simulink model "H250Model2019b"  (R2019b)
settings: Solver=ode4  StartTime=0.0  StopTime=inf  FixedStep=Ts  RelTol=1e-3
values from neighbouring files (symbols this model uses):
  ModelFail_env_P_wind = [0 0 0]    [F450DegradedParamInit.m]    (also in H250DegradedParamInit.m; H250ModelParam4S.m; H333DegradedParamInit4S.m)
  ModelFail_motor_isEnable = 0    [F450DegradedParamInit.m]    (also in H250DegradedParamInit.m; H250ModelParam4S.m; H333DegradedParamInit4S.m)
  ModelFail_motor_kCt = [1 1 1 1 1 1 1 1]    [F450DegradedParamInit.m]    (also in H250DegradedParamInit.m; H250ModelParam4S.m; H333DegradedParamInit4S.m)
  ModelFail_motor_kTc = [1 1 1 1 1 1 1 1]    [F450DegradedParamInit.m]    (also in H250DegradedParamInit.m; H250ModelParam4S.m; H333DegradedParamInit4S.m)
  ModelFail_motor_kw = [1 1 1 1 1 1 1 1]    [F450DegradedParamInit.m]    (also in H250DegradedParamInit.m; H250ModelParam4S.m; H333DegradedParamInit4S.m)
  ModelInit_motorInitRate = 0    [F450DegradedParamInit.m]    (also in H250DegradedParamInit.m; H250ModelParam4S.m; H333DegradedParamInit4S.m)
  ModelParam_Airframe_CMP = [0 0 0]    [F450DegradedParamInit.m]    (also in H250DegradedParamInit.m; H250ModelParam4S.m; H333DegradedParamInit4S.m)
  ModelParam_Airframe_J = [0.0194 0 0;0 0.0194 0;0 0 0.0291]    [F450DegradedParamInit.m]    (also in H250DegradedParamInit.m = [0.0056 0 0;0 0.0056 0;0 0 0.0104]; H250ModelParam4S.m = [0.0056 0 0;0 0.0056 0;0 0 0.0104]; H333DegradedParamInit4S.m = [0.012 0 0;0 0.012 0;0 0 0.02])
  ModelParam_Airframe_m = 1.31    [F450DegradedParamInit.m]    (also in H250DegradedParamInit.m = 0.752; H250ModelParam4S.m = 0.752; H333DegradedParamInit4S.m = 1.13)
  ModelParam_envAltitude = 0    [F450DegradedParamInit.m]    (also in H250DegradedParamInit.m; H250ModelParam4S.m; H333DegradedParamInit4S.m)
  ModelParam_envC_d = 0.055    [F450DegradedParamInit.m]    (also in H250DegradedParamInit.m; H250ModelParam4S.m; H333DegradedParamInit4S.m)
  ModelParam_envC_md = [0.001 0.001 0.00058]    [F450DegradedParamInit.m]    (also in H250DegradedParamInit.m = [0.001 0.001 0.00040]; H250ModelParam4S.m = [0.001 0.001 0.00040]; H333DegradedParamInit4S.m = [0.001 0.001 0.0002])
  ModelParam_GPSEphFinal = 0.3    [F450DegradedParamInit.m]    (also in H250DegradedParamInit.m; H250ModelParam4S.m; H333DegradedParamInit4S.m)
  ModelParam_GPSEpvFinal = 0.4    [F450DegradedParamInit.m]    (also in H250DegradedParamInit.m; H250ModelParam4S.m; H333DegradedParamInit4S.m)
  ModelParam_GPSFix3DFix = 3    [F450DegradedParamInit.m]    (also in H250DegradedParamInit.m; H250ModelParam4S.m; H333DegradedParamInit4S.m)
  ModelParam_GPSSatsVisible = 10    [F450DegradedParamInit.m]    (also in H250DegradedParamInit.m; H250ModelParam4S.m; H333DegradedParamInit4S.m)
  ModelParam_motorCr = 842.1    [F450DegradedParamInit.m]    (also in H250DegradedParamInit.m = 0; H250ModelParam4S.m = 0; H333DegradedParamInit4S.m = 0)
  ModelParam_motorFitType = 1    [F450DegradedParamInit.m]    (also in H250DegradedParamInit.m = 2; H250ModelParam4S.m = 2; H333DegradedParamInit4S.m = 2)
  ModelParam_motorJm = 0.0000687    (= 6.87e-05)    [F450DegradedParamInit.m]    (also in H250DegradedParamInit.m = 8.8493e-06; H250ModelParam4S.m = 8.8493e-06; H333DegradedParamInit4S.m = 8.8493e-06)
  ModelParam_motorMinThr = 0.05    [F450DegradedParamInit.m]    (also in H250DegradedParamInit.m = 0.148; H250ModelParam4S.m = 0.148; H333DegradedParamInit4S.m = 0.11)
  ModelParam_motorRateCurveCoeffi = [0 0 0]    [F450DegradedParamInit.m]    (also in H250DegradedParamInit.m = [-1364 3870 -372.4]; H250ModelParam4S.m = [-2143 5113 -458.4]; H333DegradedParamInit4S.m = [-1057 2662 -94.98])
  ModelParam_motorTc = 0.0214    [F450DegradedParamInit.m]    (also in H250DegradedParamInit.m = 0.035; H250ModelParam4S.m = 0.032; H333DegradedParamInit4S.m = 0.035)
  ModelParam_motorWb = 0    [F450DegradedParamInit.m]    (also in H250DegradedParamInit.m; H250ModelParam4S.m; H333DegradedParamInit4S.m)
  ModelParam_NoiseVarAcc0 = [0.1 0.1 0.1]    [F450DegradedParamInit.m]    (also in H250DegradedParamInit.m; H250ModelParam4S.m = [0.01 0.01 0.01]; H333DegradedParamInit4S.m)
  ModelParam_NoiseVarAcc1 = [0.1 0.1 0.1]    [F450DegradedParamInit.m]    (also in H250DegradedParamInit.m; H250ModelParam4S.m = [0.01 0.01 0.01]; H333DegradedParamInit4S.m)
  ModelParam_NoiseVarGPS_P0 = [1e-5 1e-5 1e-5]    [F450DegradedParamInit.m]    (also in H250DegradedParamInit.m; H250ModelParam4S.m; H333DegradedParamInit4S.m)
  ModelParam_NoiseVarGPS_V0 = [1e-5 1e-5 1e-5]    [F450DegradedParamInit.m]    (also in H250DegradedParamInit.m; H250ModelParam4S.m; H333DegradedParamInit4S.m)
  ModelParam_NoiseVarGyro0 = [0.0005 0.0005 0.0005]    [F450DegradedParamInit.m]    (also in H250DegradedParamInit.m; H250ModelParam4S.m; H333DegradedParamInit4S.m)
  ModelParam_NoiseVarGyro1 = [0.004 0.004 0.004]    [F450DegradedParamInit.m]    (also in H250DegradedParamInit.m; H250ModelParam4S.m; H333DegradedParamInit4S.m)
  ModelParam_NoiseVarMag0 = [0.000002 0.000002 0.000002]    [F450DegradedParamInit.m]    (also in H250DegradedParamInit.m; H250ModelParam4S.m; H333DegradedParamInit4S.m)
  ModelParam_NoiseVarMag1 = [0.0001 0.0001 0.0001]    [F450DegradedParamInit.m]    (also in H250DegradedParamInit.m; H250ModelParam4S.m; H333DegradedParamInit4S.m)
  ModelParam_PositionAcc0 = [0.071  0  -0.1365]    [F450DegradedParamInit.m]    (also in H250DegradedParamInit.m; H250ModelParam4S.m; H333DegradedParamInit4S.m)
  ModelParam_PositionAcc1 = [0.071  0  -0.1365]    [F450DegradedParamInit.m]    (also in H250DegradedParamInit.m; H250ModelParam4S.m; H333DegradedParamInit4S.m)
  ModelParam_rotorCt = 1.681e-05    [F450DegradedParamInit.m]    (also in H250DegradedParamInit.m = 1.448e-06; H250ModelParam4S.m = 1.345e-06; H333DegradedParamInit4S.m = 7.586e-06)
  ModelParam_WalkNoiseVarAcc0 = [0.001 0.001 0.001]    [F450DegradedParamInit.m]    (also in H250DegradedParamInit.m; H250ModelParam4S.m; H333DegradedParamInit4S.m)
  ModelParam_WalkNoiseVarAcc1 = [0.001 0.001 0.001]    [F450DegradedParamInit.m]    (also in H250DegradedParamInit.m; H250ModelParam4S.m; H333DegradedParamInit4S.m)
  ModelParam_WalkNoiseVarGPS_P0 = [0.01 0.01 0.01]    [F450DegradedParamInit.m]    (also in H250DegradedParamInit.m; H250ModelParam4S.m = [0 0 0]; H333DegradedParamInit4S.m)
  ModelParam_WalkNoiseVarGPS_V0 = [0.01 0.01 0.01]    [F450DegradedParamInit.m]    (also in H250DegradedParamInit.m; H250ModelParam4S.m = [0 0 0]; H333DegradedParamInit4S.m)
  ModelParam_WalkNoiseVarGyro0 = [0.00004 0.00004 0.00004]    [F450DegradedParamInit.m]    (also in H250DegradedParamInit.m; H250ModelParam4S.m; H333DegradedParamInit4S.m)
  ModelParam_WalkNoiseVarGyro1 = [0.00004 0.00004 0.00004]    [F450DegradedParamInit.m]    (also in H250DegradedParamInit.m; H250ModelParam4S.m; H333DegradedParamInit4S.m)
  ModelParam_WalkNoiseVarMag0 = [0.000001 0.000001 0.000001]    [F450DegradedParamInit.m]    (also in H250DegradedParamInit.m; H250ModelParam4S.m; H333DegradedParamInit4S.m)
  ModelParam_WalkNoiseVarMag1 = [0.000001 0.000001 0.000001]    [F450DegradedParamInit.m]    (also in H250DegradedParamInit.m; H250ModelParam4S.m; H333DegradedParamInit4S.m)
  MulticopterLayoutConfig = 1    [F450DegradedParamInit.m]    (also in H250DegradedParamInit.m = 6; H250ModelParam4S.m = 7; H333DegradedParamInit4S.m = 8)
  RflySimDisplayUAVType = 3    [F450DegradedParamInit.m]    (also in H250DegradedParamInit.m; H250ModelParam4S.m; H333DegradedParamInit4S.m)
  Ts = 1/1000    (= 0.001)    [F450DegradedParamInit.m]    (also in H250DegradedParamInit.m; H250ModelParam4S.m; H333DegradedParamInit4S.m)
undefined symbols (not defined in the file or in its folder): Earth, WGS84
libraries: aerolibnav x5, aerolibtransform2 x3, sharedtransform x3, aerolibutil x2, sharedutil x1, shared6dof x1, aerolibasang x1, aerolibatmos2 x1, aerolibconvert2 x1
(part 2 of 3)

== system H250Model2019b/ESC&Motor Model/MotorNonlinearDynamic4 ==
  Throttle : Inport
  BatteryEfficiency : Inport  Port=2  Unit=V
  k_omage : Inport  Port=3
  k_Tc : Inport  Port=4
  k_ct : Inport  Port=5
  ESC_MotorSteadyState : MATLAB Function  TreatAsAtomicUnit=on  mask{MotorMinThr=MotorMinThr}
      mask prompts: MotorMinThr "Minimum Throttle"
  ModelInit_motorInitRate : Constant  Value=motorInitRate
  ModelParam_motorCr : Constant  Value=motorCr
  ModelParam_motorFitType : Constant  Value=motorFitType
  ModelParam_motorRateCurveCoeffi : Constant  Value=motorRateCurveCoeffi
  ModelParam_motorTc : Constant  Value=motorTc
  ModelParam_motorWb : Constant  Value=motorWb
  ModelParam_rotorCt : Constant  Value=rotorCt
  MotorDynamic : Subsystem
      mask Display:
      | port_label('input', 1, '\varpi_{ss}(rad/s)', 'texmode', 'on');
      | port_label('input', 2, '\varpi_{0}(rad/s)', 'texmode', 'on');
      | port_label('input', 3, 'T_{c}(s)', 'texmode', 'on');
      | port_label('output', 1, '\varpi(rad/s)', 'texmode', 'on');
  Product{,1..3} (4 alike) : Product
  Square : Math  Operator=square  SaturateOnIntegerOverflow=on
  T : Outport  Unit=N
  MotorRate : Outport  Port=2  Unit=rad/s
  wires:
  ModelParam_motorFitType/1 -> ESC_MotorSteadyState/6(MotorFitType)
  ModelParam_motorRateCurveCoeffi/1 -> ESC_MotorSteadyState/5(MotorRateCurveCoeffi)
  k_ct/1 -> Product1/2
  k_Tc/1 -> Product2/2
  k_omage/1 -> Product3/1
  Product3/1 -> MotorDynamic/1(ReferenceRate)
  Product2/1 -> MotorDynamic/3(MotorTimeConstant)
  Product1/1 -> Product/2
  BatteryEfficiency/1 -> ESC_MotorSteadyState/2(BatteryEfficiency)
  MotorDynamic/1(MotorRate) -> Square/1, MotorRate/1
  ModelParam_motorTc/1 -> Product2/1
  Square/1 -> Product/1
  ESC_MotorSteadyState/1(SteadyStateRate) -> Product3/2
  Product/1 -> T/1
  ModelParam_rotorCt/1 -> Product1/1
  ModelInit_motorInitRate/1 -> MotorDynamic/2(MotorInitRate)
  ModelParam_motorCr/1 -> ESC_MotorSteadyState/3(Cr)
  Throttle/1 -> ESC_MotorSteadyState/1(Throttle)
  ModelParam_motorWb/1 -> ESC_MotorSteadyState/4(Ratebias)

== system H250Model2019b/ESC&Motor Model/MotorNonlinearDynamic5 ==
  Throttle : Inport
  BatteryEfficiency : Inport  Port=2  Unit=V
  k_omage : Inport  Port=3
  k_Tc : Inport  Port=4
  k_ct : Inport  Port=5
  ESC_MotorSteadyState : MATLAB Function  TreatAsAtomicUnit=on  mask{MotorMinThr=MotorMinThr}
      mask prompts: MotorMinThr "Minimum Throttle"
  ModelInit_motorInitRate : Constant  Value=motorInitRate
  ModelParam_motorCr : Constant  Value=motorCr
  ModelParam_motorFitType : Constant  Value=motorFitType
  ModelParam_motorRateCurveCoeffi : Constant  Value=motorRateCurveCoeffi
  ModelParam_motorTc : Constant  Value=motorTc
  ModelParam_motorWb : Constant  Value=motorWb
  ModelParam_rotorCt : Constant  Value=rotorCt
  MotorDynamic : Subsystem
      mask Display:
      | port_label('input', 1, '\varpi_{ss}(rad/s)', 'texmode', 'on');
      | port_label('input', 2, '\varpi_{0}(rad/s)', 'texmode', 'on');
      | port_label('input', 3, 'T_{c}(s)', 'texmode', 'on');
      | port_label('output', 1, '\varpi(rad/s)', 'texmode', 'on');
  Product{,1..3} (4 alike) : Product
  Square : Math  Operator=square  SaturateOnIntegerOverflow=on
  T : Outport  Unit=N
  MotorRate : Outport  Port=2  Unit=rad/s
  wires:
  ModelParam_motorWb/1 -> ESC_MotorSteadyState/4(Ratebias)
  Throttle/1 -> ESC_MotorSteadyState/1(Throttle)
  ModelParam_motorCr/1 -> ESC_MotorSteadyState/3(Cr)
  ModelInit_motorInitRate/1 -> MotorDynamic/2(MotorInitRate)
  ModelParam_rotorCt/1 -> Product1/1
  Product/1 -> T/1
  ESC_MotorSteadyState/1(SteadyStateRate) -> Product3/2
  Square/1 -> Product/1
  ModelParam_motorTc/1 -> Product2/1
  MotorDynamic/1(MotorRate) -> MotorRate/1, Square/1
  BatteryEfficiency/1 -> ESC_MotorSteadyState/2(BatteryEfficiency)
  Product1/1 -> Product/2
  Product2/1 -> MotorDynamic/3(MotorTimeConstant)
  Product3/1 -> MotorDynamic/1(ReferenceRate)
  k_omage/1 -> Product3/1
  k_Tc/1 -> Product2/2
  k_ct/1 -> Product1/2
  ModelParam_motorRateCurveCoeffi/1 -> ESC_MotorSteadyState/5(MotorRateCurveCoeffi)
  ModelParam_motorFitType/1 -> ESC_MotorSteadyState/6(MotorFitType)

== system H250Model2019b/ESC&Motor Model/MotorNonlinearDynamic6 ==
  Throttle : Inport
  BatteryEfficiency : Inport  Port=2  Unit=V
  k_omage : Inport  Port=3
  k_Tc : Inport  Port=4
  k_ct : Inport  Port=5
  ESC_MotorSteadyState : MATLAB Function  TreatAsAtomicUnit=on  mask{MotorMinThr=MotorMinThr}
      mask prompts: MotorMinThr "Minimum Throttle"
  ModelInit_motorInitRate : Constant  Value=motorInitRate
  ModelParam_motorCr : Constant  Value=motorCr
  ModelParam_motorFitType : Constant  Value=motorFitType
  ModelParam_motorRateCurveCoeffi : Constant  Value=motorRateCurveCoeffi
  ModelParam_motorTc : Constant  Value=motorTc
  ModelParam_motorWb : Constant  Value=motorWb
  ModelParam_rotorCt : Constant  Value=rotorCt
  MotorDynamic : Subsystem
      mask Display:
      | port_label('input', 1, '\varpi_{ss}(rad/s)', 'texmode', 'on');
      | port_label('input', 2, '\varpi_{0}(rad/s)', 'texmode', 'on');
      | port_label('input', 3, 'T_{c}(s)', 'texmode', 'on');
      | port_label('output', 1, '\varpi(rad/s)', 'texmode', 'on');
  Product{,1..3} (4 alike) : Product
  Square : Math  Operator=square  SaturateOnIntegerOverflow=on
  T : Outport  Unit=N
  MotorRate : Outport  Port=2  Unit=rad/s
  wires:
  ModelParam_motorFitType/1 -> ESC_MotorSteadyState/6(MotorFitType)
  ModelParam_motorRateCurveCoeffi/1 -> ESC_MotorSteadyState/5(MotorRateCurveCoeffi)
  k_ct/1 -> Product1/2
  k_Tc/1 -> Product2/2
  k_omage/1 -> Product3/1
  Product3/1 -> MotorDynamic/1(ReferenceRate)
  Product2/1 -> MotorDynamic/3(MotorTimeConstant)
  Product1/1 -> Product/2
  BatteryEfficiency/1 -> ESC_MotorSteadyState/2(BatteryEfficiency)
  MotorDynamic/1(MotorRate) -> Square/1, MotorRate/1
  ModelParam_motorTc/1 -> Product2/1
  Square/1 -> Product/1
  ESC_MotorSteadyState/1(SteadyStateRate) -> Product3/2
  Product/1 -> T/1
  ModelParam_rotorCt/1 -> Product1/1
  ModelInit_motorInitRate/1 -> MotorDynamic/2(MotorInitRate)
  ModelParam_motorCr/1 -> ESC_MotorSteadyState/3(Cr)
  Throttle/1 -> ESC_MotorSteadyState/1(Throttle)
  ModelParam_motorWb/1 -> ESC_MotorSteadyState/4(Ratebias)

== system H250Model2019b/ESC&Motor Model/MotorNonlinearDynamic7 ==
  Throttle : Inport
  BatteryEfficiency : Inport  Port=2  Unit=V
  k_omage : Inport  Port=3
  k_Tc : Inport  Port=4
  k_ct : Inport  Port=5
  ESC_MotorSteadyState : MATLAB Function  TreatAsAtomicUnit=on  mask{MotorMinThr=MotorMinThr}
      mask prompts: MotorMinThr "Minimum Throttle"
  ModelInit_motorInitRate : Constant  Value=motorInitRate
  ModelParam_motorCr : Constant  Value=motorCr
  ModelParam_motorFitType : Constant  Value=motorFitType
  ModelParam_motorRateCurveCoeffi : Constant  Value=motorRateCurveCoeffi
  ModelParam_motorTc : Constant  Value=motorTc
  ModelParam_motorWb : Constant  Value=motorWb
  ModelParam_rotorCt : Constant  Value=rotorCt
  MotorDynamic : Subsystem
      mask Display:
      | port_label('input', 1, '\varpi_{ss}(rad/s)', 'texmode', 'on');
      | port_label('input', 2, '\varpi_{0}(rad/s)', 'texmode', 'on');
      | port_label('input', 3, 'T_{c}(s)', 'texmode', 'on');
      | port_label('output', 1, '\varpi(rad/s)', 'texmode', 'on');
  Product{,1..3} (4 alike) : Product
  Square : Math  Operator=square  SaturateOnIntegerOverflow=on
  T : Outport  Unit=N
  MotorRate : Outport  Port=2  Unit=rad/s
  wires:
  ModelParam_motorWb/1 -> ESC_MotorSteadyState/4(Ratebias)
  Throttle/1 -> ESC_MotorSteadyState/1(Throttle)
  ModelParam_motorCr/1 -> ESC_MotorSteadyState/3(Cr)
  ModelInit_motorInitRate/1 -> MotorDynamic/2(MotorInitRate)
  ModelParam_rotorCt/1 -> Product1/1
  Product/1 -> T/1
  ESC_MotorSteadyState/1(SteadyStateRate) -> Product3/2
  Square/1 -> Product/1
  ModelParam_motorTc/1 -> Product2/1
  MotorDynamic/1(MotorRate) -> MotorRate/1, Square/1
  BatteryEfficiency/1 -> ESC_MotorSteadyState/2(BatteryEfficiency)
  Product1/1 -> Product/2
  Product2/1 -> MotorDynamic/3(MotorTimeConstant)
  Product3/1 -> MotorDynamic/1(ReferenceRate)
  k_omage/1 -> Product3/1
  k_Tc/1 -> Product2/2
  k_ct/1 -> Product1/2
  ModelParam_motorRateCurveCoeffi/1 -> ESC_MotorSteadyState/5(MotorRateCurveCoeffi)
  ModelParam_motorFitType/1 -> ESC_MotorSteadyState/6(MotorFitType)

== system H250Model2019b/ESC&Motor Model/MotorNonlinearDynamic8 ==
  Throttle : Inport
  BatteryEfficiency : Inport  Port=2  Unit=V
  k_omage : Inport  Port=3
  k_Tc : Inport  Port=4
  k_ct : Inport  Port=5
  ESC_MotorSteadyState : MATLAB Function  TreatAsAtomicUnit=on  mask{MotorMinThr=MotorMinThr}
      mask prompts: MotorMinThr "Minimum Throttle"
  ModelInit_motorInitRate : Constant  Value=motorInitRate
  ModelParam_motorCr : Constant  Value=motorCr
  ModelParam_motorFitType : Constant  Value=motorFitType
  ModelParam_motorRateCurveCoeffi : Constant  Value=motorRateCurveCoeffi
  ModelParam_motorTc : Constant  Value=motorTc
  ModelParam_motorWb : Constant  Value=motorWb
  ModelParam_rotorCt : Constant  Value=rotorCt
  MotorDynamic : Subsystem
      mask Display:
      | port_label('input', 1, '\varpi_{ss}(rad/s)', 'texmode', 'on');
      | port_label('input', 2, '\varpi_{0}(rad/s)', 'texmode', 'on');
      | port_label('input', 3, 'T_{c}(s)', 'texmode', 'on');
      | port_label('output', 1, '\varpi(rad/s)', 'texmode', 'on');
  Product{,1..3} (4 alike) : Product
  Square : Math  Operator=square  SaturateOnIntegerOverflow=on
  T : Outport  Unit=N
  MotorRate : Outport  Port=2  Unit=rad/s
  wires:
  ModelParam_motorFitType/1 -> ESC_MotorSteadyState/6(MotorFitType)
  ModelParam_motorRateCurveCoeffi/1 -> ESC_MotorSteadyState/5(MotorRateCurveCoeffi)
  k_ct/1 -> Product1/2
  k_Tc/1 -> Product2/2
  k_omage/1 -> Product3/1
  Product3/1 -> MotorDynamic/1(ReferenceRate)
  Product2/1 -> MotorDynamic/3(MotorTimeConstant)
  Product1/1 -> Product/2
  BatteryEfficiency/1 -> ESC_MotorSteadyState/2(BatteryEfficiency)
  MotorDynamic/1(MotorRate) -> Square/1, MotorRate/1
  ModelParam_motorTc/1 -> Product2/1
  Square/1 -> Product/1
  ESC_MotorSteadyState/1(SteadyStateRate) -> Product3/2
  Product/1 -> T/1
  ModelParam_rotorCt/1 -> Product1/1
  ModelInit_motorInitRate/1 -> MotorDynamic/2(MotorInitRate)
  ModelParam_motorCr/1 -> ESC_MotorSteadyState/3(Cr)
  Throttle/1 -> ESC_MotorSteadyState/1(Throttle)
  ModelParam_motorWb/1 -> ESC_MotorSteadyState/4(Ratebias)

== system H250Model2019b/Environment Model/Ground Model ==
  m : Inport
  g : Inport  Port=2
  wb : Inport  Port=3
  Xe : Inport  Port=4
  Ve : Inport  Port=5
  EulerAng : Inport  Port=6
  DCM : Inport  Port=7
  TerrainZ : Inport  Port=8
  Direction Cosine Matrix to Quaternions : sharedtransform/Direction Cosine Matrix  to Quaternions  aMode=0  action=None  tolerance=eps(2)
      settings: SourceProductBaseCode=AE,PW,MT,UV,VE,VP
  Direction Cosine Matrix to Quaternions1 : sharedtransform/Direction Cosine Matrix  to Quaternions  aMode=aMode  action=None  tolerance=eps(2)
      settings: SourceProductBaseCode=AE,PW,MT,UV,VE,VP
  Euler to DCM : aerolibtransform2/Wind Angles to  Direction Cosine Matrix
      settings: SourceProductBaseCode=AE
  Ground Model : MATLAB Function  TreatAsAtomicUnit=on
  OnGroundFaceup : MATLAB Function  TreatAsAtomicUnit=on
  Product : Product  Multiplication=Matrix(*)
  Product1 : Product
  Quaternion Inverse : aerolibutil/Quaternion Inverse
  Quaternion Multiplication : aerolibutil/Quaternion Multiplication
  Terminator1 : Terminator
  F_Ground : Outport
  M_Ground : Outport  Port=2
  landed : Outport  Port=3
  wires:
  Xe/1 -> Ground Model/3(Xe)
  TerrainZ/1 -> Ground Model/6(terrainZ)
  OnGroundFaceup/1(y) -> Euler to DCM/1
  Ground Model/4(takeoff) -> Terminator1/1
  Direction Cosine Matrix to Quaternions1/1 -> Quaternion Inverse/1
  Quaternion Inverse/1 -> Quaternion Multiplication/1
  Direction Cosine Matrix to Quaternions/1 -> Quaternion Multiplication/2
  Ground Model/3(landed) -> landed/1
  Quaternion Multiplication/1 -> Ground Model/5(Quet)
  Ground Model/1(F1) -> Product/2
  Euler to DCM/1 -> Direction Cosine Matrix to Quaternions1/1
  Product1/1 -> Ground Model/1(mg)
  m/1 -> Product1/1
  Ground Model/2(M1) -> M_Ground/1
  wb/1 -> Ground Model/2(wb)
  Ve/1 -> Ground Model/4(Ve)
  g/1 -> Product1/2
  EulerAng/1 -> OnGroundFaceup/1(EulerAng)
  Product/1 -> F_Ground/1
  DCM/1 -> Direction Cosine Matrix to Quaternions/1, Product/1

== system H250Model2019b/Force and Moment Model/Allocation Model ==
  index : Inport
  MotorForces : Inport  Port=2
  Wb : Inport  Port=3
  o_m : Inport  Port=4
  MotorRate : Inport  Port=5
  3x3 Cross Product : sharedutil/3x3 Cross Product  aMode=aMode
      settings: SourceProductBaseCode=AE,PW,MT,UV,VE,VP
  Assignment : Assignment  IndexMode=Zero-based  DiagnosticForDimensions=Warning  IndexOptions=Index vector (dialog)  Indices=2  OutputSizes=1
  Constant : Constant  Value=[0;0;0]
  Demux : Demux  Outputs=[3 3]
  Efficiency Function : MATLAB Function  TreatAsAtomicUnit=on
  Gain : Gain  Gain=ModelParam_motorJm
  MatrixMultiply : Product  Multiplication=Matrix(*)
  MatrixMultiply1 : Product  Multiplication=Matrix(*)
  Reshape : Reshape  OutputDimensionality=Column vector (2-D)
  F : Outport
  M : Outport  Port=2
  M_G : Outport  Port=3
  wires:
  Demux/2 -> M/1
  MatrixMultiply/1 -> Demux/1
  MotorForces/1 -> MatrixMultiply/2
  Efficiency Function/1(EfficiencyMatrix) -> MatrixMultiply/1
  Demux/1 -> F/1
  o_m/1 -> Efficiency Function/2(o_m)
  index/1 -> Efficiency Function/1(index)
  Efficiency Function/2(RotorDirectionVector) -> MatrixMultiply1/1
  MotorRate/1 -> Reshape/1
  Constant/1 -> Assignment/1
  MatrixMultiply1/1 -> Gain/1
  Reshape/1 -> MatrixMultiply1/2
  Gain/1 -> Assignment/2
  Assignment/1 -> 3x3 Cross Product/2
  Wb/1 -> 3x3 Cross Product/1
  3x3 Cross Product/1 -> M_G/1

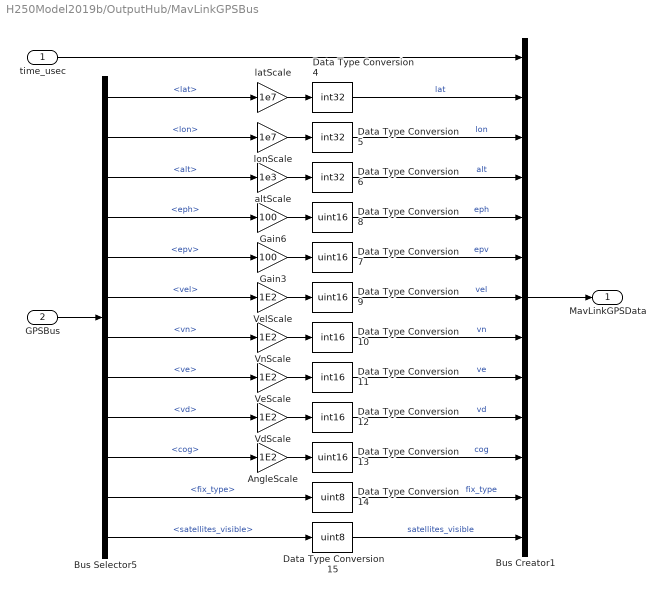
== system H250Model2019b/OutputHub/MavLinkGPSBus ==
  time_usec : Inport
  GPSBus : Inport  Port=2
  AngleScale : Gain  Gain=1E2
  Bus Creator1 : BusCreator  Inputs=13  OutDataTypeStr=Bus: MavLinkGPS  NonVirtualBus=on
  Bus Selector5 : BusSelector  OutputSignals=lat,lon,alt,eph,epv,vel,vn,ve,vd,cog,fix_type,satellites_visible
  Data Type Conversion10 : DataTypeConversion  OutDataTypeStr=int16  RndMeth=Round
  Data Type Conversion11 : DataTypeConversion  OutDataTypeStr=int16  RndMeth=Round
  Data Type Conversion12 : DataTypeConversion  OutDataTypeStr=int16  RndMeth=Round
  Data Type Conversion{7..9,13} (4 alike) : DataTypeConversion  OutDataTypeStr=uint16  RndMeth=Round
  Data Type Conversion14 : DataTypeConversion  OutDataTypeStr=uint8  RndMeth=Round
  Data Type Conversion15 : DataTypeConversion  OutDataTypeStr=uint8  RndMeth=Round
  Data Type Conversion4 : DataTypeConversion  OutDataTypeStr=int32
  Data Type Conversion5 : DataTypeConversion  OutDataTypeStr=int32
  Data Type Conversion6 : DataTypeConversion  OutDataTypeStr=int32
  Gain3 : Gain  Gain=100
  Gain6 : Gain  Gain=100
  VdScale : Gain  Gain=1E2
  VeScale : Gain  Gain=1E2
  VelScale : Gain  Gain=1E2
  VnScale : Gain  Gain=1E2
  altScale : Gain  Gain=1e3
  latScale : Gain  Gain=1e7
  lonScale : Gain  Gain=1e7
  MavLinkGPSData : Outport
  wires:
  Data Type Conversion8/1 -> Bus Creator1/5  "eph"
  Bus Selector5/5 -> Gain3/1  "<epv>"
  Bus Selector5/7 -> VnScale/1  "<vn>"
  Bus Selector5/2 -> lonScale/1  "<lon>"
  Data Type Conversion7/1 -> Bus Creator1/6  "epv"
  Data Type Conversion4/1 -> Bus Creator1/2  "lat"
  Gain3/1 -> Data Type Conversion7/1
  altScale/1 -> Data Type Conversion6/1
  Gain6/1 -> Data Type Conversion8/1
  lonScale/1 -> Data Type Conversion5/1
  VelScale/1 -> Data Type Conversion9/1
  AngleScale/1 -> Data Type Conversion13/1
  VnScale/1 -> Data Type Conversion10/1
  Bus Selector5/12 -> Data Type Conversion15/1  "<satellites_visible>"
  Bus Selector5/4 -> Gain6/1  "<eph>"
  VeScale/1 -> Data Type Conversion11/1
  Data Type Conversion13/1 -> Bus Creator1/11  "cog"
  GPSBus/1 -> Bus Selector5/1
  Bus Selector5/8 -> VeScale/1  "<ve>"
  Bus Selector5/9 -> VdScale/1  "<vd>"
  Bus Selector5/3 -> altScale/1  "<alt>"
  Data Type Conversion9/1 -> Bus Creator1/7  "vel"
  Bus Creator1/1 -> MavLinkGPSData/1
  VdScale/1 -> Data Type Conversion12/1
  time_usec/1 -> Bus Creator1/1
  Data Type Conversion10/1 -> Bus Creator1/8  "vn"
  Data Type Conversion11/1 -> Bus Creator1/9  "ve"
  Bus Selector5/11 -> Data Type Conversion14/1  "<fix_type>"
  Bus Selector5/10 -> AngleScale/1  "<cog>"
  latScale/1 -> Data Type Conversion4/1
  Data Type Conversion12/1 -> Bus Creator1/10  "vd"
  Bus Selector5/6 -> VelScale/1  "<vel>"
  Bus Selector5/1 -> latScale/1  "<lat>"
  Data Type Conversion14/1 -> Bus Creator1/12  "fix_type"
  Data Type Conversion15/1 -> Bus Creator1/13  "satellites_visible"
  Data Type Conversion5/1 -> Bus Creator1/3  "lon"
  Data Type Conversion6/1 -> Bus Creator1/4  "alt"

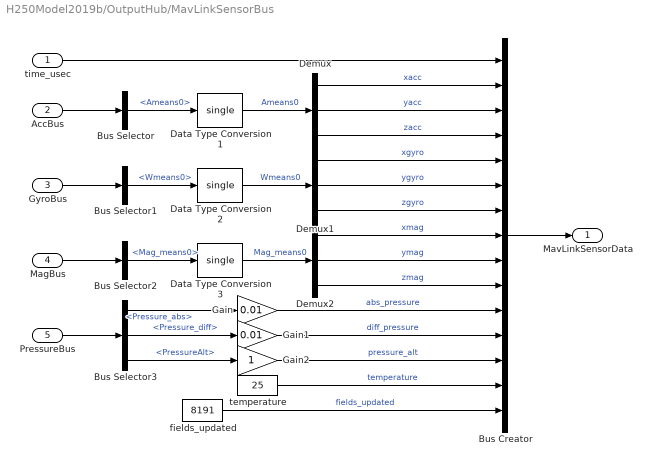
== system H250Model2019b/OutputHub/MavLinkSensorBus ==
  time_usec : Inport
  AccBus : Inport  Port=2
  GyroBus : Inport  Port=3
  MagBus : Inport  Port=4
  PressureBus : Inport  Port=5
  Bus Creator : BusCreator  Inputs=15  OutDataTypeStr=Bus: MavLinkSensor  NonVirtualBus=on
  Bus Selector : BusSelector  OutputSignals=Ameans0
  Bus Selector1 : BusSelector  OutputSignals=Wmeans0
  Bus Selector2 : BusSelector  OutputSignals=Mag_means0
  Bus Selector3 : BusSelector  OutputSignals=Pressure_abs,Pressure_diff,PressureAlt
  Data Type Conversion1 : DataTypeConversion  OutDataTypeStr=single
  Data Type Conversion2 : DataTypeConversion  OutDataTypeStr=single
  Data Type Conversion3 : DataTypeConversion  OutDataTypeStr=single
  Demux : Demux  Outputs=3
  Demux1 : Demux  Outputs=3
  Demux2 : Demux  Outputs=3
  Gain : Gain  Gain=0.01  OutDataTypeStr=single
  Gain1 : Gain  Gain=0.01  OutDataTypeStr=single
  Gain2 : Gain  OutDataTypeStr=single
  fields_updated : Constant  Value=8191  OutDataTypeStr=uint32
  temperature : Constant  Value=25  OutDataTypeStr=single
  MavLinkSensorData : Outport
  wires:
  Demux2/3 -> Bus Creator/10  "zmag"
  Gain/1 -> Bus Creator/11  "abs_pressure"
  Demux/3 -> Bus Creator/4  "zacc"
  Bus Selector/1 -> Data Type Conversion1/1  "<Ameans0>"
  Data Type Conversion3/1 -> Demux2/1  "Mag_means0"
  Demux2/2 -> Bus Creator/9  "ymag"
  Bus Selector3/2 -> Gain1/1  "<Pressure_diff>"
  Data Type Conversion1/1 -> Demux/1  "Ameans0"
  AccBus/1 -> Bus Selector/1
  MagBus/1 -> Bus Selector2/1
  Demux/2 -> Bus Creator/3  "yacc"
  Demux2/1 -> Bus Creator/8  "xmag"
  Bus Selector1/1 -> Data Type Conversion2/1  "<Wmeans0>"
  GyroBus/1 -> Bus Selector1/1
  Data Type Conversion2/1 -> Demux1/1  "Wmeans0"
  Demux1/2 -> Bus Creator/6  "ygyro"
  Bus Selector3/1 -> Gain/1  "<Pressure_abs>"
  Bus Selector2/1 -> Data Type Conversion3/1  "<Mag_means0>"
  Gain2/1 -> Bus Creator/13  "pressure_alt"
  Gain1/1 -> Bus Creator/12  "diff_pressure"
  Bus Selector3/3 -> Gain2/1  "<PressureAlt>"
  PressureBus/1 -> Bus Selector3/1
  fields_updated/1 -> Bus Creator/15  "fields_updated"
  Demux/1 -> Bus Creator/2  "xacc"
  Demux1/3 -> Bus Creator/7  "zgyro"
  temperature/1 -> Bus Creator/14  "temperature"
  Demux1/1 -> Bus Creator/5  "xgyro"
  time_usec/1 -> Bus Creator/1
  Bus Creator/1 -> MavLinkSensorData/1

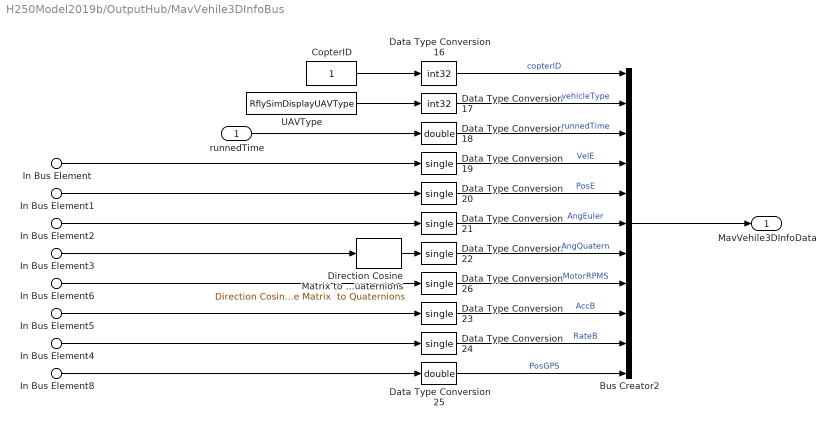
== system H250Model2019b/OutputHub/MavVehile3DInfoBus ==
  runnedTime : Inport
  In Bus Element : Inport  Port=2  PortName=Kinematics 6DOF Bus  Element=Ve
  In Bus Element1 : Inport  Port=2  PortName=Kinematics 6DOF Bus  Element=Xe
  In Bus Element2 : Inport  Port=2  PortName=Kinematics 6DOF Bus  Element=Euler
  In Bus Element3 : Inport  Port=2  PortName=Kinematics 6DOF Bus  Element=DCM
  In Bus Element4 : Inport  Port=2  PortName=Kinematics 6DOF Bus  Element=Wb
  In Bus Element5 : Inport  Port=2  PortName=Kinematics 6DOF Bus  Element=Abb
  In Bus Element6 : Inport  Port=3  PortName=Force and Moment Model Bus  Element=Motor_RPM
  In Bus Element8 : Inport  Port=4  PortName=Environment Model Bus  Element=PosGPS
  Bus Creator2 : BusCreator  Inputs=11  OutDataTypeStr=Bus: MavVehileInfo  NonVirtualBus=on
  CopterID : Constant
  Data Type Conversion16 : DataTypeConversion  OutDataTypeStr=int32
  Data Type Conversion17 : DataTypeConversion  OutDataTypeStr=int32
  Data Type Conversion18 : DataTypeConversion  OutDataTypeStr=double
  Data Type Conversion{19..24,26} (7 alike) : DataTypeConversion  OutDataTypeStr=single
  Data Type Conversion25 : DataTypeConversion  OutDataTypeStr=double
  Direction Cosine Matrix to Quaternions : sharedtransform/Direction Cosine Matrix  to Quaternions  aMode=aMode  action=None  tolerance=eps(2)
      settings: SourceProductBaseCode=AE,PW,MT,UV,VE,VP
  UAVType : Constant  Value=RflySimDisplayUAVType
  MavVehile3DInfoData : Outport
  wires:
  runnedTime/1 -> Data Type Conversion18/1
  Data Type Conversion19/1 -> Bus Creator2/4  "VelE"
  UAVType/1 -> Data Type Conversion17/1
  Data Type Conversion22/1 -> Bus Creator2/7  "AngQuatern"
  Data Type Conversion16/1 -> Bus Creator2/1  "copterID"
  Data Type Conversion17/1 -> Bus Creator2/2  "vehicleType"
  Data Type Conversion18/1 -> Bus Creator2/3  "runnedTime"
  Data Type Conversion20/1 -> Bus Creator2/5  "PosE"
  Data Type Conversion26/1 -> Bus Creator2/8  "MotorRPMS"
  Data Type Conversion25/1 -> Bus Creator2/11  "PosGPS"
  In Bus Element/1 -> Data Type Conversion19/1
  Data Type Conversion24/1 -> Bus Creator2/10  "RateB"
  In Bus Element6/1 -> Data Type Conversion26/1
  Data Type Conversion21/1 -> Bus Creator2/6  "AngEuler"
  In Bus Element4/1 -> Data Type Conversion24/1
  In Bus Element5/1 -> Data Type Conversion23/1
  CopterID/1 -> Data Type Conversion16/1
  In Bus Element1/1 -> Data Type Conversion20/1
  Data Type Conversion23/1 -> Bus Creator2/9  "AccB"
  Direction Cosine Matrix to Quaternions/1 -> Data Type Conversion22/1
  Bus Creator2/1 -> MavVehile3DInfoData/1
  In Bus Element3/1 -> Direction Cosine Matrix to Quaternions/1
  In Bus Element2/1 -> Data Type Conversion21/1
  In Bus Element8/1 -> Data Type Conversion25/1

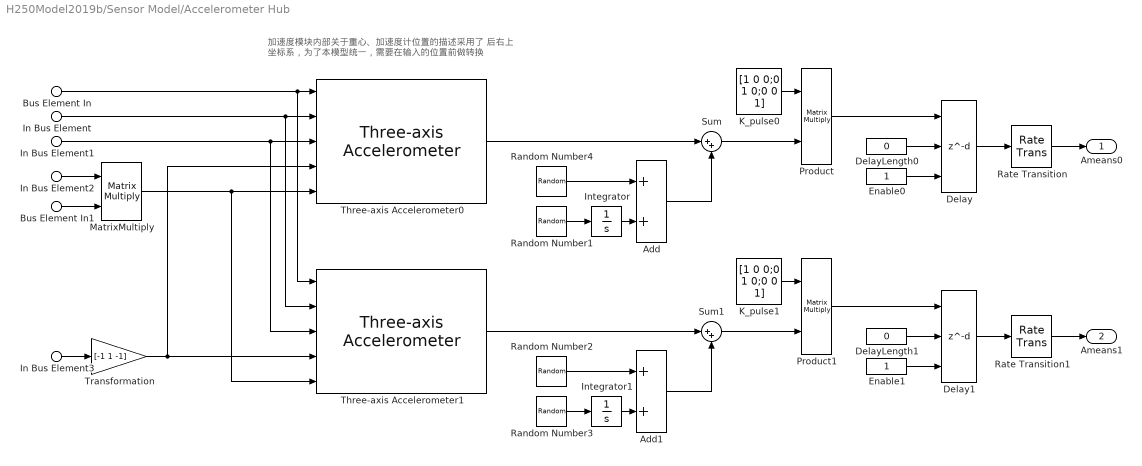
== system H250Model2019b/Sensor Model/Accelerometer Hub ==
  note: 加速度模块内部关于重心、加速度计位置的描述采用了 后右上 坐标系，为了本模型统一，需要在输入的位置前做转换
  Bus Element In1 : Inport  PortName=Environment Model Bus  Element=g
  Bus Element In : Inport  Port=2  PortName=Kinematics 6DOF Bus  Element=Abe
  In Bus Element : Inport  Port=2  PortName=Kinematics 6DOF Bus  Element=Wb
  In Bus Element1 : Inport  Port=2  PortName=Kinematics 6DOF Bus  Element=dWb
  In Bus Element2 : Inport  Port=2  PortName=Kinematics 6DOF Bus  Element=DCM
  In Bus Element3 : Inport  Port=3  PortName=Airframe Model Bus  Element=CMP
  Add : Sum
  Add1 : Sum
  Delay : Delay  DelayLengthSource=Input port  ShowEnablePort=on
      settings: InputPortMap=u0,p1,e6
  Delay1 : Delay  DelayLengthSource=Input port  ShowEnablePort=on
      settings: InputPortMap=u0,p1,e6
  DelayLength0 : Constant  Value=0
  DelayLength1 : Constant  Value=0
  Enable0 : Constant
  Enable1 : Constant
  Integrator : Integrator
  Integrator1 : Integrator
  K_pulse0 : Constant  Value=[1 0 0;0 1 0;0 0 1]
  K_pulse1 : Constant  Value=[1 0 0;0 1 0;0 0 1]
  MatrixMultiply : Product  Multiplication=Matrix(*)
  Product : Product  Multiplication=Matrix(*)
  Product1 : Product  Multiplication=Matrix(*)
  Random Number1 : RandomNumber  Mean=[0 0 0]  Variance=ModelParam_WalkNoiseVarAcc0  Seed=[233 561 6486]  SampleTime=Ts
  Random Number2 : RandomNumber  Mean=[0 0 0]  Variance=ModelParam_NoiseVarAcc1  Seed=[235 341 569]  SampleTime=Ts
  Random Number3 : RandomNumber  Mean=[0 0 0]  Variance=ModelParam_WalkNoiseVarAcc1  Seed=[3341 365 597]  SampleTime=Ts
  Random Number4 : RandomNumber  Mean=[0 0 0]  Variance=ModelParam_NoiseVarAcc0  Seed=[2331 645 9489]  SampleTime=Ts
  Rate Transition : RateTransition
  Rate Transition1 : RateTransition
  Sum : Sum  Inputs=|++
  Sum1 : Sum  Inputs=|++
  Three-axis Accelerometer0 : aerolibnav/Three-axis Accelerometer  units=Metric (MKS)  acc=[-1 1 -1].*ModelParam_PositionAcc0  gtype=on  dtype_a=on  w_a=190  z_a=0.707  a_sf_cc=[1 0 0; 0 1 0; 0 0 1]  a_bias=[0 0 0]  a_Ts=0  a_rand=off  a_seeds=[23093 23094 23095]  a_pow=[0.001 0.001 0.001]  a_sat="[-inf  -inf  -inf  inf inf inf]"
      settings: SourceProductBaseCode=AE
  Three-axis Accelerometer1 : aerolibnav/Three-axis Accelerometer  units=Metric (MKS)  acc=[-1 1 -1].*ModelParam_PositionAcc1  gtype=on  dtype_a=on  w_a=190  z_a=0.707  a_sf_cc=[1 0 0; 0 1 0; 0 0 1]  a_bias=[0 0 0]  a_Ts=0  a_rand=off  a_seeds=[23093 23094 23095]  a_pow=[0.001 0.001 0.001]  a_sat="[-inf  -inf  -inf  inf inf inf]"
      settings: SourceProductBaseCode=AE
  Transformation : Gain  Gain=[-1 1 -1]
      settings: AttributesFormatString=|
      | Coordinate system transformation
      | to aft right above
  Ameans0 : Outport
  Ameans1 : Outport  Port=2
  wires:
  MatrixMultiply/1 -> Three-axis Accelerometer0/5, Three-axis Accelerometer1/5
  Delay/1 -> Rate Transition/1
  Three-axis Accelerometer0/1 -> Sum/1
  Rate Transition/1 -> Ameans0/1
  Enable0/1 -> Delay/3
  DelayLength0/1 -> Delay/2
  DelayLength1/1 -> Delay1/2
  Enable1/1 -> Delay1/3
  Rate Transition1/1 -> Ameans1/1
  Three-axis Accelerometer1/1 -> Sum1/1
  Delay1/1 -> Rate Transition1/1
  In Bus Element1/1 -> Three-axis Accelerometer1/3, Three-axis Accelerometer0/3
  Bus Element In1/1 -> MatrixMultiply/2
  In Bus Element/1 -> Three-axis Accelerometer1/2, Three-axis Accelerometer0/2
  Bus Element In/1 -> Three-axis Accelerometer1/1, Three-axis Accelerometer0/1
  In Bus Element2/1 -> MatrixMultiply/1
  Random Number4/1 -> Add/1
  Integrator/1 -> Add/2
  Random Number1/1 -> Integrator/1
  Sum/1 -> Product/2
  Add/1 -> Sum/2
  Sum1/1 -> Product1/2
  Add1/1 -> Sum1/2
  Random Number3/1 -> Integrator1/1
  Integrator1/1 -> Add1/2
  Random Number2/1 -> Add1/1
  Product/1 -> Delay/1
  K_pulse0/1 -> Product/1
  Product1/1 -> Delay1/1
  K_pulse1/1 -> Product1/1
  In Bus Element3/1 -> Transformation/1
  Transformation/1 -> Three-axis Accelerometer0/4, Three-axis Accelerometer1/4

== system H250Model2019b/Sensor Model/Barometer ==
  In Bus Element : Inport  PortName=Environment Model Bus  Element=Altitude
  In Bus Element1 : Inport  PortName=Environment Model Bus  Element=V_wind_b_relative
  Add : Sum
  Dynamic Pressure : aerolibasang/Dynamic Pressure
  ISA Atmosphere Model : aerolibatmos2/ISA Atmosphere Model  custom=off  g=9.80665  gamma=1.4  R=287.0531  L=0.0065  h_trop=11000  h_strat=20000  rho0=1.225  P0=101325  T0=288.15  h0=0
  Integrator : Integrator
  K_pulse0 : Constant
  Pressure Function : MATLAB Function  Commented=on  TreatAsAtomicUnit=on
  Product : Product
  Random Number : RandomNumber  Variance=0.02  Seed=[23341]  SampleTime=Ts
  Random Number1 : RandomNumber  Variance=0.002  Seed=[23341]  SampleTime=Ts
  Sum : Sum  Inputs=|++
  Temperature Conversion : aerolibconvert2/Temperature Conversion  IU=K  OU=C
      settings: SourceProductBaseCode=AE
  Terminator : Terminator
  Terminator1 : Terminator
  Terminator2 : Terminator  Commented=on
  Pressure : Outport
  PressureAlt : Outport  Port=2
  diff_pressure : Outport  Port=3
  wires:
  Pressure Function/1(p) -> Terminator2/1
  Product/1 -> PressureAlt/1, Pressure Function/1(h), ISA Atmosphere Model/1
  ISA Atmosphere Model/2 -> Terminator/1
  ISA Atmosphere Model/1 -> Temperature Conversion/1
  In Bus Element/1 -> Sum/1
  Add/1 -> Sum/2
  Temperature Conversion/1 -> Terminator1/1
  Random Number/1 -> Add/1
  Integrator/1 -> Add/2
  Random Number1/1 -> Integrator/1
  Sum/1 -> Product/2
  K_pulse0/1 -> Product/1
  In Bus Element1/1 -> Dynamic Pressure/1
  ISA Atmosphere Model/4 -> Dynamic Pressure/2
  Dynamic Pressure/1 -> diff_pressure/1
  ISA Atmosphere Model/3 -> Pressure/1

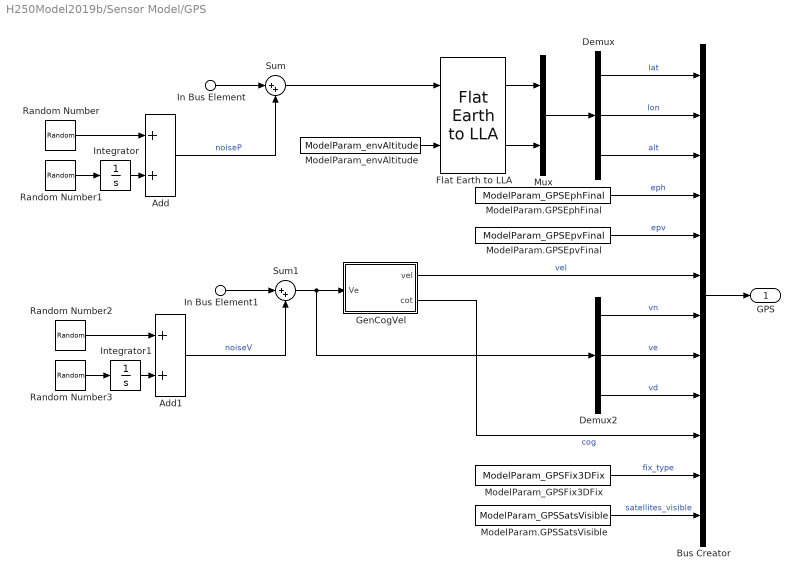
== system H250Model2019b/Sensor Model/GPS ==
  In Bus Element : Inport  PortName=Kinematics 6DOF Bus  Element=Xe
  In Bus Element1 : Inport  PortName=Kinematics 6DOF Bus  Element=Ve
  Add : Sum
  Add1 : Sum
  Bus Creator : BusCreator  Inputs=12
  Demux : Demux  Outputs=3
  Demux2 : Demux  Outputs=3
  Flat Earth to LLA : aerolibtransform2/Flat Earth to LLA  units=Metric (MKS)  ptype=Earth (WGS84)  F=1/298.257223563  R=6378137  LL0=ModelParam_GPSLatLong  psi=0
  GenCogVel : MATLAB Function  TreatAsAtomicUnit=on
  Integrator : Integrator
  Integrator1 : Integrator
  ModelParam.GPSEphFinal : Constant  Value=ModelParam_GPSEphFinal
  ModelParam.GPSEpvFinal : Constant  Value=ModelParam_GPSEpvFinal
  ModelParam.GPSSatsVisible : Constant  Value=ModelParam_GPSSatsVisible
  ModelParam_GPSFix3DFix : Constant  Value=ModelParam_GPSFix3DFix
  ModelParam_envAltitude : Constant  Value=ModelParam_envAltitude
  Mux : Mux  Inputs=2
  Random Number : RandomNumber  Mean=[0 0 0]  Variance=ModelParam_NoiseVarGPS_P0  Seed=[11 22 33]  SampleTime=Ts
  Random Number1 : RandomNumber  Mean=[0 0 0]  Variance=ModelParam_WalkNoiseVarGPS_P0  Seed=[989 656 623]  SampleTime=Ts
  Random Number2 : RandomNumber  Mean=[0 0 0]  Variance=ModelParam_NoiseVarGPS_V0  Seed=[31 52 13]  SampleTime=Ts
  Random Number3 : RandomNumber  Mean=[0 0 0]  Variance=ModelParam_WalkNoiseVarGPS_V0  Seed=[929 56 423]  SampleTime=Ts
  Sum : Sum  Inputs=|++
  Sum1 : Sum  Inputs=|++
  GPS : Outport
  wires:
  ModelParam_envAltitude/1 -> Flat Earth to LLA/2
  In Bus Element/1 -> Sum/1
  Sum/1 -> Flat Earth to LLA/1
  Random Number/1 -> Add/1
  Flat Earth to LLA/1 -> Mux/1
  Flat Earth to LLA/2 -> Mux/2
  Mux/1 -> Demux/1
  Random Number1/1 -> Integrator/1
  Integrator/1 -> Add/2
  Add/1 -> Sum/2  "noiseP"
  In Bus Element1/1 -> Sum1/1
  Add1/1 -> Sum1/2  "noiseV"
  Integrator1/1 -> Add1/2
  Random Number3/1 -> Integrator1/1
  Random Number2/1 -> Add1/1
  Sum1/1 -> Demux2/1, GenCogVel/1(Ve)
  Bus Creator/1 -> GPS/1
  Demux/1 -> Bus Creator/1  "lat"
  Demux/2 -> Bus Creator/2  "lon"
  Demux/3 -> Bus Creator/3  "alt"
  ModelParam.GPSEphFinal/1 -> Bus Creator/4  "eph"
  ModelParam.GPSEpvFinal/1 -> Bus Creator/5  "epv"
  GenCogVel/1(vel) -> Bus Creator/6  "vel"
  Demux2/1 -> Bus Creator/7  "vn"
  Demux2/2 -> Bus Creator/8  "ve"
  Demux2/3 -> Bus Creator/9  "vd"
  GenCogVel/2(cot) -> Bus Creator/10  "cog"
  ModelParam_GPSFix3DFix/1 -> Bus Creator/11  "fix_type"
  ModelParam.GPSSatsVisible/1 -> Bus Creator/12  "satellites_visible"

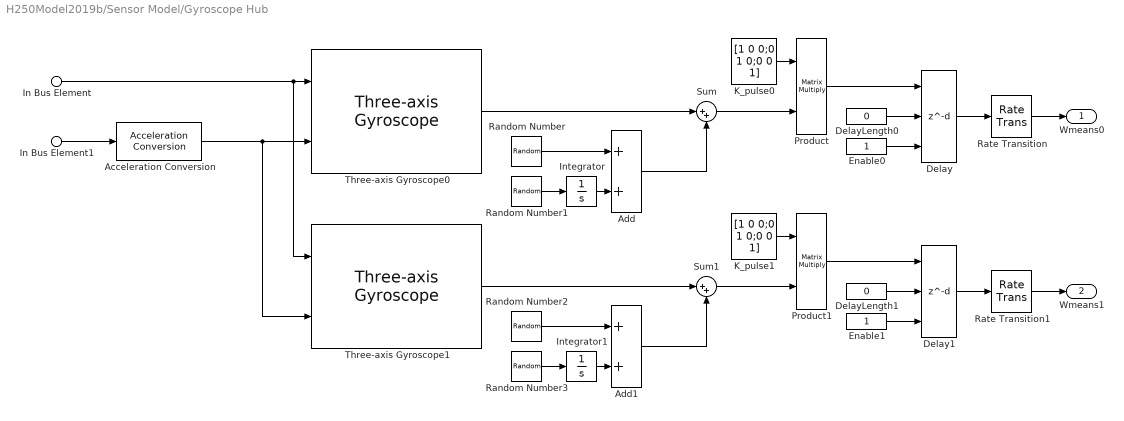
== system H250Model2019b/Sensor Model/Gyroscope Hub ==
  In Bus Element : Inport  PortName=Kinematics 6DOF Bus  Element=Wb
  In Bus Element1 : Inport  PortName=Kinematics 6DOF Bus  Element=Abe
  Acceleration Conversion : aerolibnav/Three-axis Inertial Measurement Unit/Acceleration Conversion  SystemSampleTime=-1  Latency=0  AutoFrameSizeCalculation=off
      settings: SourceProductBaseCode=AE
  Add : Sum
  Add1 : Sum
  Delay : Delay  DelayLengthSource=Input port  ShowEnablePort=on
      settings: InputPortMap=u0,p1,e6
  Delay1 : Delay  DelayLengthSource=Input port  ShowEnablePort=on
      settings: InputPortMap=u0,p1,e6
  DelayLength0 : Constant  Value=0
  DelayLength1 : Constant  Value=0
  Enable0 : Constant
  Enable1 : Constant
  Integrator : Integrator
  Integrator1 : Integrator
  K_pulse0 : Constant  Value=[1 0 0;0 1 0;0 0 1]
  K_pulse1 : Constant  Value=[1 0 0;0 1 0;0 0 1]
  Product : Product  Multiplication=Matrix(*)
  Product1 : Product  Multiplication=Matrix(*)
  Random Number : RandomNumber  Mean=[0 0 0]  Variance=ModelParam_NoiseVarGyro0  Seed=[233 541 213]  SampleTime=Ts
  Random Number1 : RandomNumber  Mean=[0 0 0]  Variance=ModelParam_WalkNoiseVarGyro0  Seed=[123 321 258]  SampleTime=Ts
  Random Number2 : RandomNumber  Mean=[0 0 0]  Variance=ModelParam_NoiseVarGyro1  Seed=[987 456 321]  SampleTime=Ts
  Random Number3 : RandomNumber  Mean=[0 0 0]  Variance=ModelParam_WalkNoiseVarGyro1  Seed=[691 147 369]  SampleTime=Ts
  Rate Transition : RateTransition
  Rate Transition1 : RateTransition
  Sum : Sum  Inputs=|++
  Sum1 : Sum  Inputs=|++
  Three-axis Gyroscope0 : aerolibnav/Three-axis Gyroscope  dtype_g=on  w_g=190  z_g=0.707  g_sf_cc=[1 0 0; 0 1 0; 0 0 1]  g_bias=[0 0 0]  g_sen=[0 0 0]  g_Ts=0  g_rand=off  g_seeds=[23093 23094 23095]  g_pow=[0.0001 0.0001 0.0001]  g_sat="[-inf  -inf  -inf  inf inf inf]"
      settings: SourceProductBaseCode=AE
  Three-axis Gyroscope1 : aerolibnav/Three-axis Gyroscope  dtype_g=on  w_g=190  z_g=0.707  g_sf_cc=[1 0 0; 0 1 0; 0 0 1]  g_bias=[0 0 0]  g_sen=[0 0 0]  g_Ts=0  g_rand=off  g_seeds=[23093 23094 23095]  g_pow=[0.0001 0.0001 0.0001]  g_sat="[-inf  -inf  -inf  inf inf inf]"
      settings: SourceProductBaseCode=AE
  Wmeans0 : Outport
  Wmeans1 : Outport  Port=2
  wires:
  In Bus Element1/1 -> Acceleration Conversion/1
  In Bus Element/1 -> Three-axis Gyroscope1/1, Three-axis Gyroscope0/1
  Acceleration Conversion/1 -> Three-axis Gyroscope0/2, Three-axis Gyroscope1/2
  Three-axis Gyroscope1/1 -> Sum1/1
  Enable0/1 -> Delay/3
  Enable1/1 -> Delay1/3
  Three-axis Gyroscope0/1 -> Sum/1
  Delay/1 -> Rate Transition/1
  Rate Transition/1 -> Wmeans0/1
  DelayLength1/1 -> Delay1/2
  Delay1/1 -> Rate Transition1/1
  Rate Transition1/1 -> Wmeans1/1
  DelayLength0/1 -> Delay/2
  Random Number/1 -> Add/1
  Integrator/1 -> Add/2
  Random Number1/1 -> Integrator/1
  Sum/1 -> Product/2
  Add/1 -> Sum/2
  Sum1/1 -> Product1/2
  Add1/1 -> Sum1/2
  Random Number3/1 -> Integrator1/1
  Integrator1/1 -> Add1/2
  Random Number2/1 -> Add1/1
  K_pulse0/1 -> Product/1
  Product/1 -> Delay/1
  Product1/1 -> Delay1/1
  K_pulse1/1 -> Product1/1

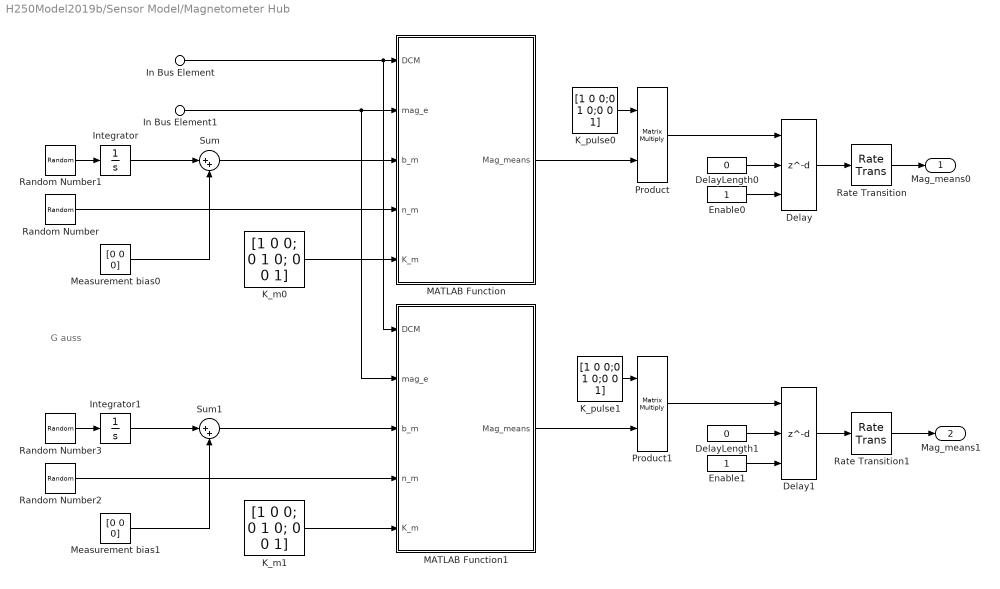
== system H250Model2019b/Sensor Model/Magnetometer Hub ==
  note: G auss
  In Bus Element : Inport  PortName=Kinematics 6DOF Bus  Element=DCM
  In Bus Element1 : Inport  Port=2  PortName=Environment Model Bus  Element=mag_e
  Delay : Delay  DelayLengthSource=Input port  ShowEnablePort=on
      settings: InputPortMap=u0,p1,e6
  Delay1 : Delay  DelayLengthSource=Input port  ShowEnablePort=on
      settings: InputPortMap=u0,p1,e6
  DelayLength0 : Constant  Value=0
  DelayLength1 : Constant  Value=0
  Enable0 : Constant
  Enable1 : Constant
  Integrator : Integrator
  Integrator1 : Integrator
  K_m0 : Constant  Value=[1 0 0; 0 1 0; 0 0 1]
  K_m1 : Constant  Value=[1 0 0; 0 1 0; 0 0 1]
  K_pulse0 : Constant  Value=[1 0 0;0 1 0;0 0 1]
  K_pulse1 : Constant  Value=[1 0 0;0 1 0;0 0 1]
  MATLAB Function : MATLAB Function  TreatAsAtomicUnit=on
  MATLAB Function1 : MATLAB Function  TreatAsAtomicUnit=on
  Measurement bias0 : Constant  Value=[0 0 0]
  Measurement bias1 : Constant  Value=[0 0 0]
  Product : Product  Multiplication=Matrix(*)
  Product1 : Product  Multiplication=Matrix(*)
  Random Number : RandomNumber  Mean=[0 0 0]  Variance=ModelParam_NoiseVarMag0  Seed=[156 489 756]  SampleTime=Ts
  Random Number1 : RandomNumber  Mean=[0 0 0]  Variance=ModelParam_WalkNoiseVarMag0  Seed=[159 753 654]  SampleTime=Ts
  Random Number2 : RandomNumber  Mean=[0 0 0]  Variance=ModelParam_NoiseVarMag1  Seed=[666 588 477]  SampleTime=Ts
  Random Number3 : RandomNumber  Mean=[0 0 0]  Variance=ModelParam_WalkNoiseVarMag1  Seed=[111 222 333]  SampleTime=Ts
  Rate Transition : RateTransition
  Rate Transition1 : RateTransition
  Sum : Sum  Inputs=|++
  Sum1 : Sum  Inputs=|++
  Mag_means0 : Outport
  Mag_means1 : Outport  Port=2
  wires:
  In Bus Element1/1 -> MATLAB Function/2(mag_e), MATLAB Function1/2(mag_e)
  In Bus Element/1 -> MATLAB Function1/1(DCM), MATLAB Function/1(DCM)
  K_m0/1 -> MATLAB Function/5(K_m)
  Integrator/1 -> Sum/1
  Random Number/1 -> MATLAB Function/4(n_m)
  K_m1/1 -> MATLAB Function1/5(K_m)
  Integrator1/1 -> Sum1/1
  Random Number2/1 -> MATLAB Function1/4(n_m)
  Rate Transition/1 -> Mag_means0/1
  Delay/1 -> Rate Transition/1
  DelayLength0/1 -> Delay/2
  Enable0/1 -> Delay/3
  MATLAB Function/1(Mag_means) -> Product/2
  MATLAB Function1/1(Mag_means) -> Product1/2
  Enable1/1 -> Delay1/3
  DelayLength1/1 -> Delay1/2
  Delay1/1 -> Rate Transition1/1
  Rate Transition1/1 -> Mag_means1/1
  Random Number1/1 -> Integrator/1
  Random Number3/1 -> Integrator1/1
  Product/1 -> Delay/1
  K_pulse0/1 -> Product/1
  K_pulse1/1 -> Product1/1
  Product1/1 -> Delay1/1
  Sum/1 -> MATLAB Function/3(b_m)
  Measurement bias0/1 -> Sum/2
  Sum1/1 -> MATLAB Function1/3(b_m)
  Measurement bias1/1 -> Sum1/2

== system H250Model2019b/ESC&Motor Model/MotorNonlinearDynamic1/MotorDynamic ==
  ReferenceRate : Inport  Unit=rad/s
  MotorInitRate : Inport  Port=2  Unit=rad/s
  MotorTimeConstant : Inport  Port=3  Unit=s
  Divide : Product  Inputs=*/
  Integrator : Integrator  InitialConditionSource=external
  Sum : Sum  Inputs=-+|
  MotorRate : Outport  Unit=rad/s
  wires:
  ReferenceRate/1 -> Sum/2
  Sum/1 -> Divide/1
  MotorTimeConstant/1 -> Divide/2
  Divide/1 -> Integrator/1
  Integrator/1 -> MotorRate/1, Sum/1
  MotorInitRate/1 -> Integrator/2

== system H250Model2019b/ESC&Motor Model/MotorNonlinearDynamic2/MotorDynamic ==
  ReferenceRate : Inport  Unit=rad/s
  MotorInitRate : Inport  Port=2  Unit=rad/s
  MotorTimeConstant : Inport  Port=3  Unit=s
  Divide : Product  Inputs=*/
  Integrator : Integrator  InitialConditionSource=external
  Sum : Sum  Inputs=-+|
  MotorRate : Outport  Unit=rad/s
  wires:
  MotorInitRate/1 -> Integrator/2
  Integrator/1 -> Sum/1, MotorRate/1
  Divide/1 -> Integrator/1
  MotorTimeConstant/1 -> Divide/2
  Sum/1 -> Divide/1
  ReferenceRate/1 -> Sum/2

== system H250Model2019b/ESC&Motor Model/MotorNonlinearDynamic3/MotorDynamic ==
  ReferenceRate : Inport  Unit=rad/s
  MotorInitRate : Inport  Port=2  Unit=rad/s
  MotorTimeConstant : Inport  Port=3  Unit=s
  Divide : Product  Inputs=*/
  Integrator : Integrator  InitialConditionSource=external
  Sum : Sum  Inputs=-+|
  MotorRate : Outport  Unit=rad/s
  wires:
  ReferenceRate/1 -> Sum/2
  Sum/1 -> Divide/1
  MotorTimeConstant/1 -> Divide/2
  Divide/1 -> Integrator/1
  Integrator/1 -> MotorRate/1, Sum/1
  MotorInitRate/1 -> Integrator/2

== system H250Model2019b/ESC&Motor Model/MotorNonlinearDynamic4/MotorDynamic ==
  ReferenceRate : Inport  Unit=rad/s
  MotorInitRate : Inport  Port=2  Unit=rad/s
  MotorTimeConstant : Inport  Port=3  Unit=s
  Divide : Product  Inputs=*/
  Integrator : Integrator  InitialConditionSource=external
  Sum : Sum  Inputs=-+|
  MotorRate : Outport  Unit=rad/s
  wires:
  MotorInitRate/1 -> Integrator/2
  Integrator/1 -> Sum/1, MotorRate/1
  Divide/1 -> Integrator/1
  MotorTimeConstant/1 -> Divide/2
  Sum/1 -> Divide/1
  ReferenceRate/1 -> Sum/2

== system H250Model2019b/ESC&Motor Model/MotorNonlinearDynamic5/MotorDynamic ==
  ReferenceRate : Inport  Unit=rad/s
  MotorInitRate : Inport  Port=2  Unit=rad/s
  MotorTimeConstant : Inport  Port=3  Unit=s
  Divide : Product  Inputs=*/
  Integrator : Integrator  InitialConditionSource=external
  Sum : Sum  Inputs=-+|
  MotorRate : Outport  Unit=rad/s
  wires:
  ReferenceRate/1 -> Sum/2
  Sum/1 -> Divide/1
  MotorTimeConstant/1 -> Divide/2
  Divide/1 -> Integrator/1
  Integrator/1 -> MotorRate/1, Sum/1
  MotorInitRate/1 -> Integrator/2

== system H250Model2019b/ESC&Motor Model/MotorNonlinearDynamic6/MotorDynamic ==
  ReferenceRate : Inport  Unit=rad/s
  MotorInitRate : Inport  Port=2  Unit=rad/s
  MotorTimeConstant : Inport  Port=3  Unit=s
  Divide : Product  Inputs=*/
  Integrator : Integrator  InitialConditionSource=external
  Sum : Sum  Inputs=-+|
  MotorRate : Outport  Unit=rad/s
  wires:
  MotorInitRate/1 -> Integrator/2
  Integrator/1 -> Sum/1, MotorRate/1
  Divide/1 -> Integrator/1
  MotorTimeConstant/1 -> Divide/2
  Sum/1 -> Divide/1
  ReferenceRate/1 -> Sum/2

== system H250Model2019b/ESC&Motor Model/MotorNonlinearDynamic7/MotorDynamic ==
  ReferenceRate : Inport  Unit=rad/s
  MotorInitRate : Inport  Port=2  Unit=rad/s
  MotorTimeConstant : Inport  Port=3  Unit=s
  Divide : Product  Inputs=*/
  Integrator : Integrator  InitialConditionSource=external
  Sum : Sum  Inputs=-+|
  MotorRate : Outport  Unit=rad/s
  wires:
  ReferenceRate/1 -> Sum/2
  Sum/1 -> Divide/1
  MotorTimeConstant/1 -> Divide/2
  Divide/1 -> Integrator/1
  Integrator/1 -> MotorRate/1, Sum/1
  MotorInitRate/1 -> Integrator/2

== system H250Model2019b/ESC&Motor Model/MotorNonlinearDynamic8/MotorDynamic ==
  ReferenceRate : Inport  Unit=rad/s
  MotorInitRate : Inport  Port=2  Unit=rad/s
  MotorTimeConstant : Inport  Port=3  Unit=s
  Divide : Product  Inputs=*/
  Integrator : Integrator  InitialConditionSource=external
  Sum : Sum  Inputs=-+|
  MotorRate : Outport  Unit=rad/s
  wires:
  MotorInitRate/1 -> Integrator/2
  Integrator/1 -> Sum/1, MotorRate/1
  Divide/1 -> Integrator/1
  MotorTimeConstant/1 -> Divide/2
  Sum/1 -> Divide/1
  ReferenceRate/1 -> Sum/2

== matlab function H250Model2019b/Sensor Model/GPS/GenCogVel ==
  data: vel output; Ve input; cot output
function [vel,cot] = Ang360(Ve)
vel=norm(Ve(1:2));

if vel < 1
    cot = 0;
else
    cot=atan2d(Ve(2),Ve(1));
end
 
if cot<0
    cot=cot+360;
end
